simulink model "TurtleBotZeroDynamic"  (R2022b)
settings: Solver=FixedStepAuto  StartTime=0.0  StopTime=inf  RelTol=1e-3
StartFcn:
  | % Path del Blocco di cui vogliamo estrarre gli output
  | blk = 'TurtleBotZeroDynamic/Subscriber Odometria/Subsystem';
  | 
  | % Si allega al blocco in questione un event listener che esegue la funzione 'displayBusdata'
  | % in occasione dell'evento 'PostOutputs' ossia quando sono disponibili nuovi output dal blocco blk
  | h = add_exec_event_listener(blk, 'PostOutputs', @displayBusdata);
StopFcn:
  | pause(0.1);
  | if out.controllo_attivo.Data
  | 
  |      rng("shuffle");
  |      node_name = strcat("NODO_STOP_",num2str(randi([1000,9999])));
  |      fprintf("CREAZIONE %s\n",node_name);
  |      nodo = ros2node(node_name);
  | 
  |      pause(0.5)    % Permette la scrittura del segnale 'Scelta' nel workspace con il nome di 'scelta_turtlebot'
  | 
  |      if out.scelta_turtlebot.Data == 1
  |           disp('FERMO TURTLE 1')
  |           [pub, msg] = ros2publisher(nodo,'/turtle1/cmd_vel','geometry_msgs/Twist','Depth',1);
  |           %disp(pub)
  |       elseif out.scelta_turtlebot.Data == 2
  |           disp('FERMO TURTLE 2')
  |           [pub, msg] = ros2publisher(nodo,'/turtle2/cmd_vel','geometry_msgs/Twist','Depth',1);
  |           %disp(pub)
  |       elseif out.scelta_turtlebot.Data == 3
  |           disp('FERMO TURTLE 3')
  |           [pub, msg] = ros2publisher(nodo,'/turtle3/cmd_vel','geometry_msgs/Twist','Depth',1);
  |           %disp(pub)
  |      end
  | 
  |      %pause(1)
  | 
  |      send(pub,msg);
  | 
  |      pause(1);
  | 
  |      %delete(nodo);
  | 
  |  end
  | 
  |  % Do not delete, this is an auto-generated function to log ROS 2 message.
  |  ros.slros.internal.ROSUtil.logROSMessageToBagFile(bdroot);
  | 
  |  %clear all
  |  clear
model workspace (MAT data in the model file):
  ROSLoggingInfo_ : object (value not decoded)
  ROSLoggingReload_ : object (value not decoded)
  ROSLoggingTable_ : object (value not decoded)
  SL_ROS_VariableLengthArrays_MaxSizes : object (value not decoded)
undefined symbols (not defined in the file): angular, linear
libraries: ros2lib x10
(part 2 of 2)

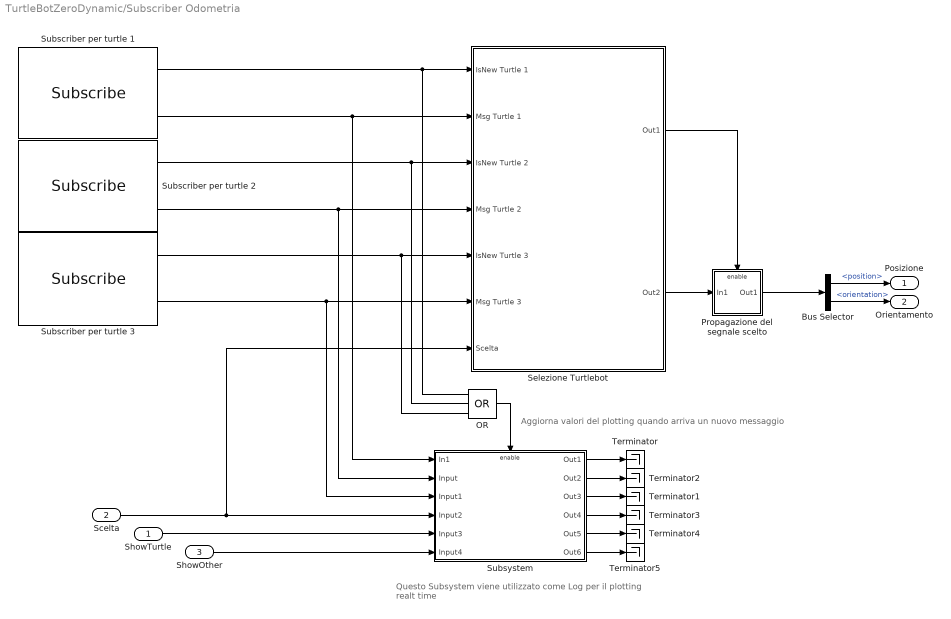
== system TurtleBotZeroDynamic/Subscriber Odometria ==
  note: Aggiorna valori del plotting quando arriva un nuovo messaggio
  note: Questo Subsystem viene utilizzato
      | come Log per il plotting realt time
  ShowTurtle : Inport
  Scelta : Inport  Port=2
  ShowOther : Inport  Port=3
  Bus Selector : BusSelector  OutputSignals=pose.pose.position,pose.pose.orientation
  OR : Logic  Operator=OR  Inputs=3  IconShape=distinctive  AllPortsSameDT=off  OutDataTypeStr=boolean
  Propagazione del segnale scelto : Subsystem  TreatAsAtomicUnit=on
  Selezione Turtlebot : Subsystem
  Subscriber per turtle 1 : ros2lib/Subscribe  topicSource=Specify your own  topic=/turtle1/odom  messageType=nav_msgs/Odometry  sampleTime=0.01  QOSHistory=Keep last  QOSDepth=1  QOSReliability=Reliable  QOSDurability=Volatile
  Subscriber per turtle 2 : ros2lib/Subscribe  topicSource=Specify your own  topic=/turtle2/odom  messageType=nav_msgs/Odometry  sampleTime=0.01  QOSHistory=Keep last  QOSDepth=1  QOSReliability=Reliable  QOSDurability=Volatile
  Subscriber per turtle 3 : ros2lib/Subscribe  topicSource=Specify your own  topic=/turtle3/odom  messageType=nav_msgs/Odometry  sampleTime=0.01  QOSHistory=Keep last  QOSDepth=1  QOSReliability=Reliable  QOSDurability=Volatile
  Subsystem : Subsystem  TreatAsAtomicUnit=on
  Terminator{,1..5} (6 alike) : Terminator
  Posizione : Outport
  Orientamento : Outport  Port=2
  wires:
  Bus Selector/1 -> Posizione/1  "<position>"
  Bus Selector/2 -> Orientamento/1  "<orientation>"
  Subscriber per turtle 1/1 -> OR/1, Selezione Turtlebot/1(IsNew Turtle 1)
  Subscriber per turtle 1/2 -> Selezione Turtlebot/2(Msg Turtle 1), Subsystem/1(In1)
  Subscriber per turtle 2/1 -> OR/2, Selezione Turtlebot/3(IsNew Turtle 2)
  Subscriber per turtle 2/2 -> Subsystem/2(Input), Selezione Turtlebot/4(Msg Turtle 2)
  Subscriber per turtle 3/1 -> OR/3, Selezione Turtlebot/5(IsNew Turtle 3)
  Subscriber per turtle 3/2 -> Subsystem/3(Input1), Selezione Turtlebot/6(Msg Turtle 3)
  ShowTurtle/1 -> Subsystem/5(Input3)
  Scelta/1 -> Selezione Turtlebot/7(Scelta), Subsystem/4(Input2)
  Selezione Turtlebot/1(Out1) -> Propagazione del segnale scelto/Enable
  Propagazione del segnale scelto/1(Out1) -> Bus Selector/1
  Selezione Turtlebot/2(Out2) -> Propagazione del segnale scelto/1(In1)
  ShowOther/1 -> Subsystem/6(Input4)
  Subsystem/1(Out1) -> Terminator/1
  Subsystem/2(Out2) -> Terminator2/1
  Subsystem/3(Out3) -> Terminator1/1
  Subsystem/4(Out4) -> Terminator3/1
  Subsystem/5(Out5) -> Terminator4/1
  Subsystem/6(Out6) -> Terminator5/1
  OR/1 -> Subsystem/Enable

== system TurtleBotZeroDynamic/BACK HOME/Controllo HOME ==
  x : Inport
  y : Inport  Port=2
  theta : Inport  Port=3
  Input : Inport  Port=4
  Controllore HOME : Subsystem
      settings: PortSchema="{\"entries\":[{\"content\":{\"sides\":[{\"content\":{\"connectorIds\":[\"In1\",\"In2\",\"In3\",\"In4\"]},\"type\":\"ConnectorPlacement.EquallySpacedRectSide\",\"uuid\":\"3398d184-1d91-4856-bdb6-081106b2fd7e\"},{\"content\":{\"connectorIds\":[\"Out1\",\"Out2\"],\"side\":\"RIGHT\"},\"type\":\"ConnectorPlacement.EquallySpacedRectSide\",\"uuid\":\"4a9b3e39-ddd1-4bc3-a041-e3c6184ce332\"},{\"content\":{\"connectorIds\":[\"In5\",\"In6\",\"In7\",\"In8\"],\"side\":\"TOP\"},\"type\":\"ConnectorPlacement.EquallySpacedRectSide\",\"uuid\":\"7222a75e-6da4-44a3-949f-633ca5d91dea\"}]},\"type\":\"ConnectorPlacement.EquallySpacedConnector\",\"uuid\":\"a2c04aa1-a248-43ff-800f-6b153036dc17\"}],\"packageUris\":[\"http://schema.mathworks.com/mf0/Connector/R2020b\"],\"version\":\"1.0\"}"
  K_5 : Constant  Value=0.5
  K_6 : Constant  Value=0.5
  x origine : Constant  Value=0
  y origine : Constant  Value=0
  Velocità Lineare : Outport
  Velocità angolare : Outport  Port=2
  wires:
  x origine/1 -> Controllore HOME/5(x_des)
  y origine/1 -> Controllore HOME/6(y_des)
  Controllore HOME/1(Velocità Lineare) -> Velocità Lineare/1
  K_6/1 -> Controllore HOME/8(K_2)
  K_5/1 -> Controllore HOME/7(K_1)
  y/1 -> Controllore HOME/2(y)
  x/1 -> Controllore HOME/1(x)
  theta/1 -> Controllore HOME/3(theta)
  Controllore HOME/2(Velocità angolare) -> Velocità angolare/1
  Input/1 -> Controllore HOME/4(Input)

== system TurtleBotZeroDynamic/Controller/M1Maker ==
  dy_desdt : Inport
  Reshape : Reshape  OutputDimensionality=Column vector (2-D)
  M1 : Outport
  wires:
  dy_desdt/1 -> Reshape/1
  Reshape/1 -> M1/1

== system TurtleBotZeroDynamic/Publish Velocità Lineare e Angolare/Selezione Publisher ==
  Msg : Inport
  Scelta : Inport  Port=2
  Abilita Controllo : Inport  Port=3
  ROS2 Publisher : MATLAB Function  TreatAsAtomicUnit=on
  wires:
  Scelta/1 -> ROS2 Publisher/2(scelta)
  Msg/1 -> ROS2 Publisher/3(Msg)
  Abilita Controllo/1 -> ROS2 Publisher/1(abilita)

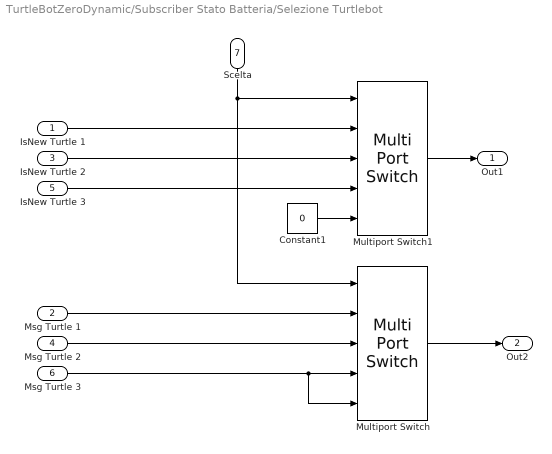
== system TurtleBotZeroDynamic/Subscriber Stato Batteria/Selezione Turtlebot ==
  IsNew Turtle 1 : Inport
  Msg Turtle 1 : Inport  Port=2
  IsNew Turtle 2 : Inport  Port=3
  Msg Turtle 2 : Inport  Port=4
  IsNew Turtle 3 : Inport  Port=5
  Msg Turtle 3 : Inport  Port=6
  Scelta : Inport  Port=7
  Constant1 : Constant  Value=0
  Multiport Switch : MultiPortSwitch  DataPortForDefault=Additional data port  SaturateOnIntegerOverflow=off  InputSameDT=off
  Multiport Switch1 : MultiPortSwitch  DataPortForDefault=Additional data port  SaturateOnIntegerOverflow=off  InputSameDT=off
  Out1 : Outport
  Out2 : Outport  Port=2
  wires:
  Constant1/1 -> Multiport Switch1/5
  IsNew Turtle 1/1 -> Multiport Switch1/2
  Msg Turtle 2/1 -> Multiport Switch/3
  IsNew Turtle 2/1 -> Multiport Switch1/3
  Msg Turtle 1/1 -> Multiport Switch/2
  Msg Turtle 3/1 -> Multiport Switch/5, Multiport Switch/4
  IsNew Turtle 3/1 -> Multiport Switch1/4
  Multiport Switch/1 -> Out2/1
  Multiport Switch1/1 -> Out1/1
  Scelta/1 -> Multiport Switch1/1, Multiport Switch/1

== system TurtleBotZeroDynamic/Subscriber Stato Batteria/Subsystem ==
  In1 : Inport
  Out1 : Outport
  wires:
  In1/1 -> Out1/1

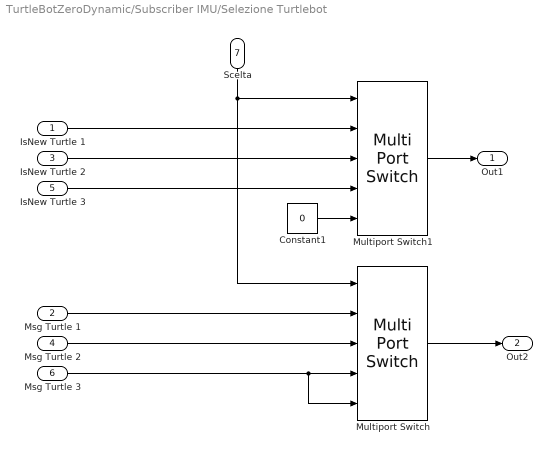
== system TurtleBotZeroDynamic/Subscriber IMU/Selezione Turtlebot ==
  IsNew Turtle 1 : Inport
  Msg Turtle 1 : Inport  Port=2
  IsNew Turtle 2 : Inport  Port=3
  Msg Turtle 2 : Inport  Port=4
  IsNew Turtle 3 : Inport  Port=5
  Msg Turtle 3 : Inport  Port=6
  Scelta : Inport  Port=7
  Constant1 : Constant  Value=0
  Multiport Switch : MultiPortSwitch  DataPortForDefault=Additional data port  SaturateOnIntegerOverflow=off  InputSameDT=off
  Multiport Switch1 : MultiPortSwitch  DataPortForDefault=Additional data port  SaturateOnIntegerOverflow=off  InputSameDT=off
  Out1 : Outport
  Out2 : Outport  Port=2
  wires:
  Constant1/1 -> Multiport Switch1/5
  IsNew Turtle 1/1 -> Multiport Switch1/2
  Msg Turtle 2/1 -> Multiport Switch/3
  IsNew Turtle 2/1 -> Multiport Switch1/3
  Msg Turtle 1/1 -> Multiport Switch/2
  Msg Turtle 3/1 -> Multiport Switch/5, Multiport Switch/4
  IsNew Turtle 3/1 -> Multiport Switch1/4
  Multiport Switch/1 -> Out2/1
  Multiport Switch1/1 -> Out1/1
  Scelta/1 -> Multiport Switch1/1, Multiport Switch/1

== system TurtleBotZeroDynamic/Subscriber IMU/Subsystem ==
  In1 : Inport
  Enable : EnablePort
  Out1 : Outport
  wires:
  In1/1 -> Out1/1

== system TurtleBotZeroDynamic/Subscriber Odometria/Propagazione del segnale scelto ==
  In1 : Inport
  Enable : EnablePort
  Out1 : Outport
  wires:
  In1/1 -> Out1/1

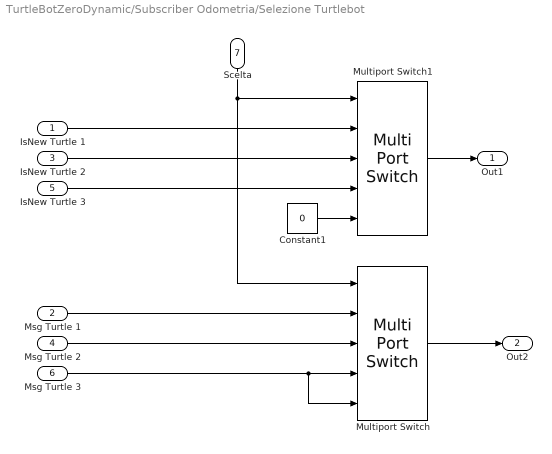
== system TurtleBotZeroDynamic/Subscriber Odometria/Selezione Turtlebot ==
  IsNew Turtle 1 : Inport
  Msg Turtle 1 : Inport  Port=2
  IsNew Turtle 2 : Inport  Port=3
  Msg Turtle 2 : Inport  Port=4
  IsNew Turtle 3 : Inport  Port=5
  Msg Turtle 3 : Inport  Port=6
  Scelta : Inport  Port=7
  Constant1 : Constant  Value=0
  Multiport Switch : MultiPortSwitch  DataPortForDefault=Additional data port  SaturateOnIntegerOverflow=off  InputSameDT=off
  Multiport Switch1 : MultiPortSwitch  DataPortForDefault=Additional data port  SaturateOnIntegerOverflow=off  InputSameDT=off
  Out1 : Outport
  Out2 : Outport  Port=2
  wires:
  Constant1/1 -> Multiport Switch1/5
  IsNew Turtle 1/1 -> Multiport Switch1/2
  Msg Turtle 2/1 -> Multiport Switch/3
  IsNew Turtle 2/1 -> Multiport Switch1/3
  Msg Turtle 1/1 -> Multiport Switch/2
  Msg Turtle 3/1 -> Multiport Switch/5, Multiport Switch/4
  IsNew Turtle 3/1 -> Multiport Switch1/4
  Multiport Switch/1 -> Out2/1
  Multiport Switch1/1 -> Out1/1
  Scelta/1 -> Multiport Switch1/1, Multiport Switch/1

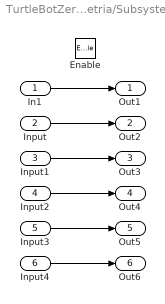
== system TurtleBotZeroDynamic/Subscriber Odometria/Subsystem ==
  In1 : Inport
  Input : Inport  Port=2
  Input1 : Inport  Port=3
  Input2 : Inport  Port=4
  Input3 : Inport  Port=5
  Input4 : Inport  Port=6
  Enable : EnablePort
  Out1 : Outport
  Out2 : Outport  Port=2
  Out3 : Outport  Port=3
  Out4 : Outport  Port=4
  Out5 : Outport  Port=5
  Out6 : Outport  Port=6
  wires:
  In1/1 -> Out1/1
  Input4/1 -> Out6/1
  Input/1 -> Out2/1
  Input1/1 -> Out3/1
  Input2/1 -> Out4/1
  Input3/1 -> Out5/1

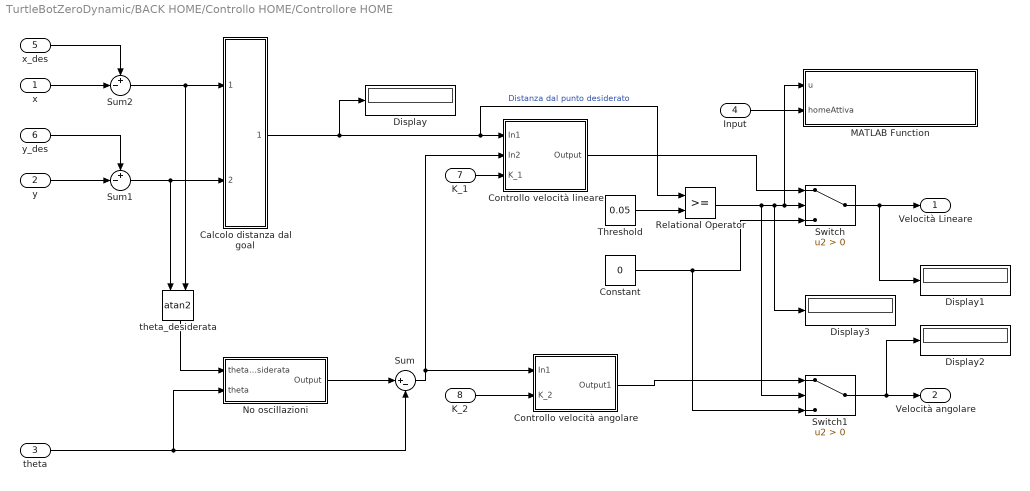
== system TurtleBotZeroDynamic/BACK HOME/Controllo HOME/Controllore HOME ==
  x : Inport
  y : Inport  Port=2
  theta : Inport  Port=3
  Input : Inport  Port=4
  x_des : Inport  Port=5
  y_des : Inport  Port=6
  K_1 : Inport  Port=7
  K_2 : Inport  Port=8
  Calcolo distanza dal goal : Subsystem
  Constant : Constant  Value=0
  Controllo velocità angolare : Subsystem
  Controllo velocità lineare : Subsystem
  Display{,1..3} (4 alike) : Display
  MATLAB Function : MATLAB Function  TreatAsAtomicUnit=on
  No oscillazioni : Subsystem
  Relational Operator : RelationalOperator  OutDataTypeStr=boolean  RndMeth=Simplest  InputSameDT=off
  Sum : Sum  Inputs=|+-
  Sum1 : Sum  Inputs=+-|
  Sum2 : Sum  Inputs=+-|
  Switch : Switch  Criteria=u2 > Threshold  SaturateOnIntegerOverflow=off  InputSameDT=off
  Switch1 : Switch  Criteria=u2 > Threshold  SaturateOnIntegerOverflow=off  InputSameDT=off
  Threshold : Constant  Value=0.05
  theta_desiderata : Trigonometry  Operator=atan2
  Velocità Lineare : Outport
  Velocità angolare : Outport  Port=2
  wires:
  x/1 -> Sum2/2
  x_des/1 -> Sum2/1
  y_des/1 -> Sum1/1
  y/1 -> Sum1/2
  Sum2/1 -> Calcolo distanza dal goal/1(e_x), theta_desiderata/2
  Sum1/1 -> Calcolo distanza dal goal/2(e_y), theta_desiderata/1
  theta/1 -> No oscillazioni/2(theta), Sum/2
  Sum/1 -> Controllo velocità lineare/2(In2), Controllo velocità angolare/1(In1)
  theta_desiderata/1 -> No oscillazioni/1(theta desiderata)
  No oscillazioni/1(Output) -> Sum/1
  Calcolo distanza dal goal/1(Out1) -> Display/1, Relational Operator/1, Controllo velocità lineare/1(In1)  "Distanza dal punto desiderato"
  Threshold/1 -> Relational Operator/2
  Relational Operator/1 -> Switch1/2, Display3/1, MATLAB Function/1(u), Switch/2
  Controllo velocità lineare/1(Output) -> Switch/1
  Switch/1 -> Display1/1, Velocità Lineare/1
  Constant/1 -> Switch1/3, Switch/3
  Controllo velocità angolare/1(Output1) -> Switch1/1
  Switch1/1 -> Display2/1, Velocità angolare/1
  K_1/1 -> Controllo velocità lineare/3(K_1)
  K_2/1 -> Controllo velocità angolare/2(K_2)
  Input/1 -> MATLAB Function/2(homeAttiva)

== system TurtleBotZeroDynamic/BACK HOME/Controllo HOME/Controllore HOME/Calcolo distanza dal goal ==
  e_x : Inport
  e_y : Inport  Port=2
  Square : Math  Operator=square
  Square Root : Sqrt
  Square1 : Math  Operator=square
  Sum2 : Sum  Inputs=+|+
  Out1 : Outport
  wires:
  Square/1 -> Sum2/1
  e_y/1 -> Square1/1  "e_y"
  Sum2/1 -> Square Root/1
  Square1/1 -> Sum2/2
  e_x/1 -> Square/1  "e_x"
  Square Root/1 -> Out1/1

== system TurtleBotZeroDynamic/BACK HOME/Controllo HOME/Controllore HOME/Controllo velocità angolare ==
  In1 : Inport
  K_2 : Inport  Port=2
  Product : Product
  Output1 : Outport
  wires:
  In1/1 -> Product/1
  Product/1 -> Output1/1
  K_2/1 -> Product/2

== system TurtleBotZeroDynamic/BACK HOME/Controllo HOME/Controllore HOME/Controllo velocità lineare ==
  In1 : Inport
  In2 : Inport  Port=2
  K_1 : Inport  Port=3
  Cos : Trigonometry  Operator=cos
  Product : Product
  Product1 : Product
  Output : Outport
  wires:
  In2/1 -> Cos/1
  Product/1 -> Output/1
  Cos/1 -> Product/2
  K_1/1 -> Product1/1
  In1/1 -> Product1/2
  Product1/1 -> Product/1

== system TurtleBotZeroDynamic/BACK HOME/Controllo HOME/Controllore HOME/No oscillazioni ==
  theta desiderata : Inport
  theta : Inport  Port=2
  " " : MATLAB Function  TreatAsAtomicUnit=on
  Memory : Memory  LinearizeAsDelay=on
  Output : Outport
  wires:
  theta desiderata/1 -> " "/1(u)
  " "/2(n_giri) -> Memory/1
  Memory/1 -> " "/3("n_giri ")
  " "/1(y) -> Output/1
  theta/1 -> " "/2(theta)

== matlab function TurtleBotZeroDynamic/Controller/Control ==
  data: A input; b input; M1 input; u1 output; M2 input; u2 output
function [u1, u2] = control(A, b, M1, M2)

    u = inv(A)*(-b + M1 + M2);

    u1 = u(1);
    u2 = u(2);
    
end

== matlab function TurtleBotZeroDynamic/BACK HOME/Controllo HOME/Controllore HOME/MATLAB Function ==
  data: u input; homeAttiva input
function isArrived(u,homeAttiva)
%{
    isArrived.m è una funzione che disattiva la modalità HOME e attiva quella STOP quando si
    raggiunge la posizione configurata come HOME.
    
    Input: 
        u:  Valore booleano che indica se il turtleBot non è giunto a destinazione o meno
    Ouput:
        None
%}

coder.extrinsic('set_param');

persistent isArrived;

if isempty(isArrived)
    isArrived = -1;
end

if u == 1 || homeAttiva == 0
    isArrived = 0;
    return
elseif u == 0 && homeAttiva == 1

    if isArrived == 0

        disp("HOME RAGGIUNTA")
        isArrived = 1;

        % SI BLOCCA IL TURTLEBOT
        %set_param('interfaccia_turtleBot/Publish Velocità Lineare e Angolare/BLOCCO', 'Value','1');

        %pause(0.1);

        % SI DISABILITA LA MODALITA HOME
        %set_param('interfaccia_turtleBot/BACK HOME/HOME', 'Value','0');

    end
   
end

end

== matlab function TurtleBotZeroDynamic/Controller/Normal Form ==
  data: L input; x input; A output; b output
function [A, b] = normalForm(L, x)
    
    A = [cos(x(3)), -L*sin(x(3));
         sin(x(3)),  L*cos(x(3))];
    
    b = [0;
         0];
    
end

== matlab function TurtleBotZeroDynamic/Publish Velocità Lineare e Angolare/Selezione Publisher/ROS2 Publisher ==
  data: abilita input; scelta input; Msg input
function fcn(abilita,scelta,Msg)

if abilita ~= 1
    disp("CONTROLLO BLOCCATO")
    return
end

coder.extrinsic('pubSetpoint');     % Necessario in quanto sono presenti funzioni non supportate dal code generator di Simulink

pubSetpoint(scelta,Msg);

end

== matlab function TurtleBotZeroDynamic/Controller/M2Maker ==
  data: x input; y_des input; c input; M2 output
function M2 = M2Maker(x, y_des, c)

    M2 = [-c(1)*(x(1) - y_des(1));
          -c(2)*(x(2) - y_des(2))];

end

== matlab function TurtleBotZeroDynamic/BACK HOME/Controllo HOME/Controllore HOME/No oscillazioni/  ==
  data: u input; theta input; y output; n_giri input; n_giri output
function [y, n_giri] = getRealAngle(u,theta,n_giri)

theta_d = u + pi*2*n_giri;

if (abs(theta_d + 2*pi - theta) < abs(theta_d - theta))

    theta_d = theta_d + 2*pi;
    n_giri = n_giri + 1;
else
    if (abs(theta_d - 2*pi - theta) < abs(theta_d - theta))

        theta_d = theta_d - 2*pi;
        n_giri = n_giri - 1;

    end
end

y = theta_d;
